simulink model "NotchFilter"  (R2021a)
settings: Solver=ode1  StartTime=0.0  StopTime=10.0  FixedStep=0.001  RelTol=1e-3
settings Model: Creator=a4327481  LastModifiedBy=a4327481

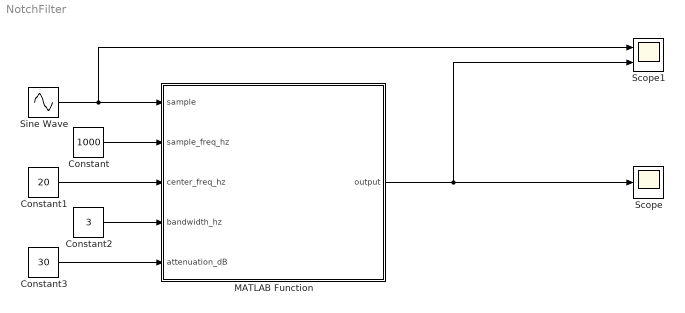
== system NotchFilter ==
  Constant : Constant  Value=1000
  Constant1 : Constant  Value=20
  Constant2 : Constant  Value=3
  Constant3 : Constant  Value=30
  MATLAB Function : MATLAB Function  TreatAsAtomicUnit=on
  Scope : Scope
  Scope1 : Scope  NumInputPorts=2
  Sine Wave : Sin  Frequency=30*2*pi  SampleTime=0
  wires:
  Sine Wave/1 -> Scope1/1, MATLAB Function/1(sample)
  Constant/1 -> MATLAB Function/2(sample_freq_hz)
  Constant1/1 -> MATLAB Function/3(center_freq_hz)
  Constant2/1 -> MATLAB Function/4(bandwidth_hz)
  Constant3/1 -> MATLAB Function/5(attenuation_dB)
  MATLAB Function/1(output) -> Scope/1, Scope1/2

== matlab function NotchFilter/MATLAB Function ==
  data: sample input; output output; sample_freq_hz input; center_freq_hz input; bandwidth_hz input; attenuation_dB input
function output = fcn( sample,sample_freq_hz,  center_freq_hz, bandwidth_hz,  attenuation_dB)

persistent ret
    if isempty(ret)
    ret=NotchFilter_init( sample_freq_hz,  center_freq_hz, bandwidth_hz,  attenuation_dB);
    end
output = NotchFilter_apply(sample,ret); 
end
